simulink model "sim_bandpower_singleBand"  (R2016b)
settings: Solver=FixedStepDiscrete  StartTime=0.0  StopTime=(size(sm_EEG_data,1)-1)/sm.p.EEG.sr  RelTol=1e-3  EnableMultiTasking=on
undefined symbols (not defined in the file): fdesignblkfcn, gcbh, sm
libraries: dspstat3 x1, dspsrcs4 x1
settings Model: Creator=ronens  LastModifiedBy=Csc
settings DataIOCC: LimitDataPoints=on  SaveFormat=Array  SignalLoggingSaveFormat=ModelDataLogs
settings OptimizationCC: ExpressionDepthLimit=2147483647  LifeSpan=inf
settings DebuggingCC: UnderspecifiedInitializationDetection=Classic  MergeDetectMultiDrivingBlocksExec=none  SolverPrmCheckMsg=warning  FcnCallInpInsideContextMsg=warning  StateNameClashWarn=warning  SFUnexpectedBacktrackingDiag=warning  SFNoUnconditionalDefaultTransitionDiag=warning  SFExecutionAtInitializationDiag=none
settings HardwareCC: ProdBitPerPointer=32  ProdBitPerSizeT=32  ProdBitPerPtrDiffT=32  ProdLargestAtomicFloat=None  ProdIntDivRoundTo=Undefined  ProdEndianess=Unspecified  ProdWordSize=32  ProdHWDeviceType=32-bit Generic
settings ModelReferenceCC: PropagateSignalLabelsOutOfModel=off
settings GRTTargetCC: TargetLangStandard=C89/C90 (ANSI)  GeneratePreprocessorConditionals=Disable all
settings ConfigComp: CovMetricSettings=dw  CovHtmlReporting=on  CovSaveCumulativeToWorkspaceVar=on  CovSaveSingleToWorkspaceVar=on  CovExternalEMLEnable=off
settings ConfigurationSet: Description=SimMechanics 2G

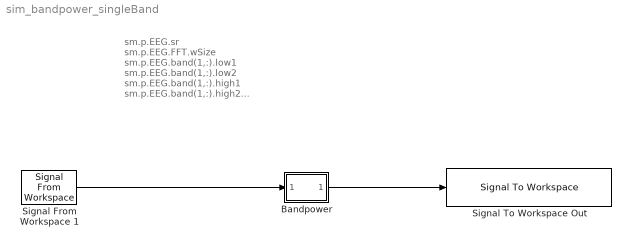
== system sim_bandpower_singleBand ==
  note: sm.p.EEG.sr
      | sm.p.EEG.FFT.wSize
      | sm.p.EEG.band(1,:).low1
      | sm.p.EEG.band(1,:).low2
      | sm.p.EEG.band(1,:).high1
      | sm.p.EEG.band(1,:).high2
      | sm.p.EEG.band_stop_dB
      | sm.p.EEG.band_pass_dB
  Bandpower : Subsystem
  Signal From Workspace 1 : dspsrcs4/Signal From Workspace  X=sm_EEG_data  Ts=1/sm.p.EEG.sr  nsamps=1  OutputAfterFinalValue=Setting to zero  ignoreOrWarnInputAndFrameLengths=off  OutputFrames=on
  Signal To Workspace Out : SignalToWorkspace  VariableName=Bandpower_singleBand
      settings: CopyFcn=dspblkcopystw(gcbh);
  wires:
  Signal From Workspace 1/1 -> Bandpower/1(In1)
  Bandpower/1(Out1) -> Signal To Workspace Out/1

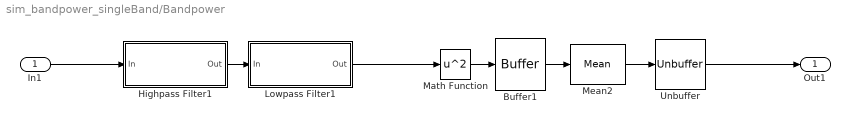
== system sim_bandpower_singleBand/Bandpower ==
  In1 : Inport
  Buffer1 : Buffer  N=sm.p.EEG.FFT.wSize  V=sm.p.EEG.FFT.wSize -1
  Highpass Filter1 : Subsystem  DialogController=fdesignblkfcn  InitFcn=fdesignblkfcn(gcbh, {'InitFcn'});  mask(Highpass Filter){}
      mask help: Design a highpass filter
      settings: CopyFcn=fdesignblkfcn(gcbh, {'CopyFcn'});
      mask Help: helpview(mapfilelocation('dsp'), 'dsphighpassfilter');
      mask Display: disp('Highpass')
  Lowpass Filter1 : Subsystem  DialogController=fdesignblkfcn  InitFcn=fdesignblkfcn(gcbh, {'InitFcn'});  mask(Lowpass Filter){}
      mask help: Design a lowpass filter
      settings: CopyFcn=fdesignblkfcn(gcbh, {'CopyFcn'});
      mask Help: helpview(mapfilelocation('dsp'), 'dsplowpassfilter');
      mask Display: disp('Lowpass')
  Math Function : Math  Operator=square  SaturateOnIntegerOverflow=on
  Mean2 : dspstat3/Mean  run=off  reset_popup=None  InputProcessing=Columns as channels (frame based)  directionMode=Each column  dimension=1  roiEnable=off  roiType=Rectangles  roiPortion=Entire ROI  roiOutput=Individual statistics for each ROI  roiFlag=off  outputMin=[]  outputMax=[]  roundingMode=Floor  overflowMode=off
  Unbuffer : Unbuffer  SampleBasedProcessing=Same as frame based
  Out1 : Outport
  wires:
  Mean2/1 -> Unbuffer/1
  Buffer1/1 -> Mean2/1
  In1/1 -> Highpass Filter1/1(In)
  Highpass Filter1/1(Out) -> Lowpass Filter1/1(In)
  Math Function/1 -> Buffer1/1
  Lowpass Filter1/1(Out) -> Math Function/1
  Unbuffer/1 -> Out1/1

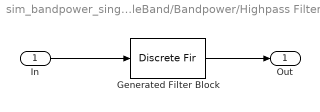
== system sim_bandpower_singleBand/Bandpower/Highpass Filter1 ==
  In : Inport
  Generated Filter Block : DiscreteFir  Tag=BlockMethodSubSystem  Coefficients=[-0.01452316881636536 0.01378332050081129 0.0086281788958850695 0.0050946801800974464 0.0023756050205232943 -2.6988064518257168e-05 -0.0023037363487080093 -0.0044845719026811353 -0.006381354903815765 -0.0077719158000679623 -0.0083616806654994626 -0.0079291798289980609 -0.0063032405073229951 -0.0034543783506806648 0.00047949263719845983 0.0051617960392515306 0.010088810021049369 0.014630750426209729 0.01812546320509744 0.019826394175360588 0.019120082529387485 0.015489839157705963 0.0087673461624230477 -0.0010930687943044306 -0.013770600647901093 -0.028597549665246341 -0.04477995329117259 -0.061199780373967574 -0.076760676726968097 -0.090304357628250356 -0.1008068118057108 -0.1074562043005536 0.89027276925589682 -0.1074562043005536 -0.1008068118057108 -0.090304357628250356 -0.076760676726968097 -0.061199780373967574 -0.04477995329117259 -0.028597549665246341 -0.013770600647901093 -0.0010930687943044306 0.0087673461624230477 0.015489839157705963 0.019120082529387485 0.019826394175360588 0.01812546320509744 0.014630750426209729 0.010088810021049369 0.0051617960392515306 0.00047949263719845983 -0.0034543783506806648 -0.0063032405073229951 -0.0079291798289980609 -0.0083616806654994626 -0.0077719158000679623 -0.006381354903815765 -0.0044845719026811353 -0.0023037363487080093 -2.6988064518257168e-05 0.0023756050205232943 0.0050946801800974464 0.0086281788958850695 0.01378332050081129 -0.01452316881636536]  InputProcessing=Columns as channels (frame based)
  Out : Outport
  wires:
  Generated Filter Block/1 -> Out/1
  In/1 -> Generated Filter Block/1

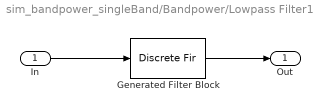
== system sim_bandpower_singleBand/Bandpower/Lowpass Filter1 ==
  In : Inport
  Generated Filter Block : DiscreteFir  Tag=BlockMethodSubSystem  Coefficients=[0.0014125794353498109 0.002331830339148553 0.0025353276339117646 0.00068273235772871603 -0.003727226834498781 -0.0097177341632059041 -0.014667777704966124 -0.015249948318767859 -0.0092793505294327915 0.0023898371240199793 0.015159617478443365 0.02208169858201052 0.01719271369813314 -0.00058431927348025648 -0.025087862791762464 -0.043870913606156581 -0.04275793202924183 -0.012373047895538634 0.04632957273771434 0.12046945051982437 0.18889352742301754 0.22992010389958362 0.22992010389958362 0.18889352742301754 0.12046945051982437 0.04632957273771434 -0.012373047895538634 -0.04275793202924183 -0.043870913606156581 -0.025087862791762464 -0.00058431927348025648 0.01719271369813314 0.02208169858201052 0.015159617478443365 0.0023898371240199793 -0.0092793505294327915 -0.015249948318767859 -0.014667777704966124 -0.0097177341632059041 -0.003727226834498781 0.00068273235772871603 0.0025353276339117646 0.002331830339148553 0.0014125794353498109]  InputProcessing=Columns as channels (frame based)
  Out : Outport
  wires:
  In/1 -> Generated Filter Block/1
  Generated Filter Block/1 -> Out/1
